simulink model "clik_transpose"  (R2024b)
settings: Solver=ode1  StartTime=0.0  StopTime=4  FixedStep=0.001  RelTol=1e-3
undefined symbols (not defined in the file or in its folder): DiscIntNeverNeededParam, q0
settings Model: Creator=Xp  LastModifiedBy=22guo
settings SolverCC: AlgebraicLoopSolver=TrustRegion
settings DataIOCC: LimitDataPoints=on  SaveFormat=Array  SignalLoggingSaveFormat=ModelDataLogs  ReturnWorkspaceOutputs=off
settings OptimizationCC: ExpressionDepthLimit=2147483647  InitFltsAndDblsToZero=on  LifeSpan=inf
settings DebuggingCC: SaveWithParameterizedLinksMsg=none  UnderspecifiedInitializationDetection=Classic  MergeDetectMultiDrivingBlocksExec=none  SolverPrmCheckMsg=warning  MultiTaskDSMMsg=warning  MultiTaskCondExecSysMsg=none  FcnCallInpInsideContextMsg=warning  UnconnectedInputMsg=warning  UnconnectedOutputMsg=warning  UnconnectedLineMsg=warning  StateNameClashWarn=warning  SFUnexpectedBacktrackingDiag=warning  SFNoUnconditionalDefaultTransitionDiag=warning  SFExecutionAtInitializationDiag=none  ArithmeticOperatorsInVariantConditions=warning
settings HardwareCC: ProdBitPerPointer=32  ProdBitPerSizeT=32  ProdBitPerPtrDiffT=32  ProdLargestAtomicFloat=None  ProdIntDivRoundTo=Undefined  ProdEndianess=Unspecified  ProdWordSize=32  ProdHWDeviceType=32-bit Generic
settings ModelReferenceCC: EnableRefExpFcnMdlSchedulingChecks=on  PropagateSignalLabelsOutOfModel=off
settings SFSimCC: CustomCodeUndefinedFunction=UseInterfaceOnly
settings RTWCC: GPUComputeCapability=3.5  DLArmComputeVersion=19.05
settings CodeAppCC: StateflowObjectComments=on
settings GRTTargetCC: TargetLangStandard=C89/C90 (ANSI)  CombineOutputUpdateFcns=off  GRTInterface=on
settings ConfigComp: CovMetricSettings=dw  CovSaveCumulativeToWorkspaceVar=on  CovSaveSingleToWorkspaceVar=on

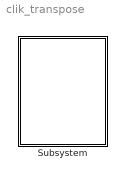
== system clik_transpose ==
  Subsystem : Subsystem

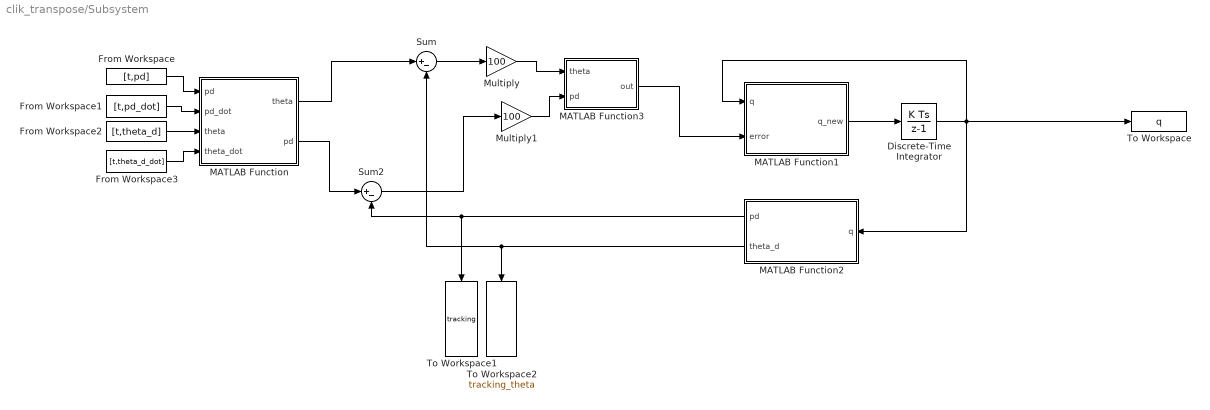
== system clik_transpose/Subsystem ==
  Discrete-Time Integrator : DiscreteIntegrator  InitialCondition=q0  SampleTime=0.001  ICPrevOutput=DiscIntNeverNeededParam  ICPrevScaledInput=DiscIntNeverNeededParam
  From Workspace : FromWorkspace  VariableName=[t,pd]  SampleTime=0.001
  From Workspace1 : FromWorkspace  VariableName=[t,pd_dot]  SampleTime=0.001
  From Workspace2 : FromWorkspace  VariableName=[t,theta_d]  SampleTime=0.001
  From Workspace3 : FromWorkspace  VariableName=[t,theta_d_dot]  SampleTime=0.001
  MATLAB Function : MATLAB Function  TreatAsAtomicUnit=on
  MATLAB Function1 : MATLAB Function  TreatAsAtomicUnit=on
  MATLAB Function2 : MATLAB Function  TreatAsAtomicUnit=on
  MATLAB Function3 : MATLAB Function  TreatAsAtomicUnit=on
  Multiply : Gain  Gain=100
  Multiply1 : Gain  Gain=100
  Sum : Sum  Inputs=|+-
  Sum2 : Sum  Inputs=|+-
  To Workspace : ToWorkspace  VariableName=q  SampleTime=-1
  To Workspace1 : ToWorkspace  VariableName=tracking  SampleTime=-1
      settings: Save2DSignal=2-D array (concatenate along first dimension)
  To Workspace2 : ToWorkspace  VariableName=tracking_theta  SampleTime=-1
      settings: Save2DSignal=2-D array (concatenate along first dimension)
  wires:
  Sum/1 -> Multiply/1
  From Workspace/1 -> MATLAB Function/1("pd ")
  From Workspace1/1 -> MATLAB Function/2(pd_dot)
  From Workspace2/1 -> MATLAB Function/3("theta ")
  From Workspace3/1 -> MATLAB Function/4(theta_dot)
  MATLAB Function3/1(out) -> MATLAB Function1/2(error)
  MATLAB Function1/1(q_new) -> Discrete-Time Integrator/1
  MATLAB Function2/1(pd) -> Sum2/2, To Workspace1/1
  MATLAB Function2/2(theta_d) -> Sum/2, To Workspace2/1
  Discrete-Time Integrator/1 -> To Workspace/1, MATLAB Function2/1(q), MATLAB Function1/1(q)
  MATLAB Function/1(theta) -> Sum/1
  Sum2/1 -> Multiply1/1
  MATLAB Function/2(pd) -> Sum2/1
  Multiply/1 -> MATLAB Function3/1(theta)
  Multiply1/1 -> MATLAB Function3/2(pd)

== matlab function clik_transpose/Subsystem/MATLAB Function1 ==
  data: q input; q_new output; error input
function q_new  = J_transpose(q,error)
[q_new]=jacobian_transpose(q,error);
end

== matlab function clik_transpose/Subsystem/MATLAB Function ==
  data: pd input; pd_dot input; theta input; theta_dot input; theta output; pd output
function [theta, pd]=data_prep(pd,pd_dot,theta,theta_dot)
pd=pd;
theta=theta;

end

== matlab function clik_transpose/Subsystem/MATLAB Function2 ==
  data: q input; pd output; theta_d output
function [pd,theta_d]= direct_k(q)
[pd, theta_d] =direct_kin(q);
end

== matlab function clik_transpose/Subsystem/MATLAB Function3 ==
  data: theta input; out output; pd input
function out = combine(theta,pd)
out=[pd;theta];
end
